simulink model "simscapeFuzzyComplete20Final"  (R2020b)
settings: Solver=FixedStepAuto  StartTime=0.0  StopTime=10  FixedStep=1e-5  RelTol=1e-1
InitFcn:
  | Param
values from neighbouring files (symbols this model uses):
  c = 3.5077E-3    (= 0.0035077)    [Param.m]
  g = 9.81    [Param.m]
  Jm = 3.2284E-3    (= 0.0032284)    [Param.m]
  K = 0.0274    [Param.m]
  L = 2.75E-3    (= 0.00275)    [Param.m]
  m = 0.051    [Param.m]
  R = 4    [Param.m]
undefined symbols (not defined in the file or in its folder): X, Y, Z
libraries: sm_lib x29, nesl_utility x10, fuzblock x2, simulink x2, pid_lib x2
(part 1 of 3)
settings Model: EnablePacing=on  Creator=HASSAN  LastModifiedBy=sara6
settings DebuggingCC: SFMachineParentedDataDiag=error
settings ExplorerConfigSet: InternalSimMechanicsExplorerSettings="<ExplorerConfiguration><canonicalview>default</canonicalview><AnimationSetting><BasePlaybackSpeed>1.0</BasePlaybackSpeed><PlaybackSpeedFactor>1.0</PlaybackSpeedFactor></AnimationSetting><TilePanel><TileInfo><Tiles Columns=\"1\" Count=\"1\" Rows=\"1\"><Column Weight=\"1\"/><Row Weight=\"1\"/><Tile Height=\"1\" Width=\"1\" X=\"0\" Y=\"0\"/></Tiles></TileInfo><SceneInfo><SceneViewer><BGColor><R>0.60000002384185791</R><G>0.60000002384185791</G><B>0.60000002384185791</B></BGColor><Camera><DoPerspective>off</DoPerspective><Position><X>0.124999998925166445</X><Y>0.0174999977718945862</Y><Z>1.04360001290421245</Z></Position><Center><X>0.124999998925166445</X><Y>0.0174999977718945862</Y><Z>0.0436000129042124485</Z></Center><Up><X>0</X><Y>1</Y><Z>-0</Z></Up><ViewLimDist>1</ViewLimDist><YLim>0.187288632229957203</YLim><XLim>0.154500006139278417</XLim></Camera></SceneViewer></SceneInfo></TilePanel><MechEditorPanel><Cameras/><GfxPanelCameraMap/><VideoCreator><PlaybackSpeedRatio>1.0</PlaybackSpeedRatio><FrameRate>30</FrameRate><VideoFormat>MPEG-4</VideoFormat><FrameSize>auto</FrameSize></VideoCreator></MechEditorPanel></ExplorerConfiguration>"

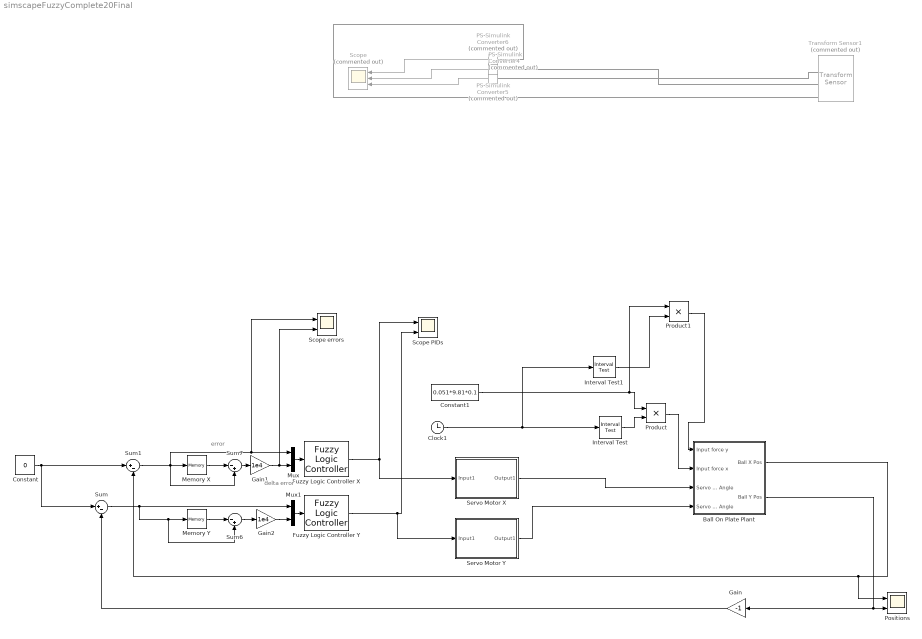
== system simscapeFuzzyComplete20Final ==
  note: delta error
  note: error
  Ball On Plate Plant : Subsystem
  Clock1 : Clock
  Constant : Constant  Value=0
  Constant1 : Constant  Value=0.051*9.81*0.1
  Fuzzy Logic Controller X : fuzblock/Fuzzy Logic  Controller  FIS='simpleFuzzy2.fis'  OutputSampleNumber=101  DataType=double  FuzzifiedInputs=off  RuleFiringStrengths=off  RuleOutputs=off  AggregatedOutputs=off  SimulateUsing=Code generation  OutOfRangeInputValueMessage=warning  NoRuleFiredMessage=warning  EmptyOutputFuzzySetMessage=warning
  Fuzzy Logic Controller Y : fuzblock/Fuzzy Logic  Controller  FIS='simpleFuzzy2.fis'  OutputSampleNumber=101  DataType=double  FuzzifiedInputs=off  RuleFiringStrengths=off  RuleOutputs=off  AggregatedOutputs=off  SimulateUsing=Code generation  OutOfRangeInputValueMessage=warning  NoRuleFiredMessage=warning  EmptyOutputFuzzySetMessage=warning
  Gain : Gain  Gain=-1
  Gain1 : Gain  Gain=1e4
  Gain2 : Gain  Gain=1e4
  Interval Test : simulink/Logic and Bit Operations/Interval Test  IntervalClosedRight=on  uplimit=0.2  IntervalClosedLeft=on  lowlimit=0.1  OutDataTypeStr=boolean
  Interval Test1 : simulink/Logic and Bit Operations/Interval Test  IntervalClosedRight=on  uplimit=0.2  IntervalClosedLeft=on  lowlimit=0.1  OutDataTypeStr=boolean
  Memory X : Memory
  Memory Y : Memory
  Mux : Mux  Inputs=2
  Mux1 : Mux  Inputs=2
  PS-Simulink Converter4 : nesl_utility/PS-Simulink Converter  Commented=on  PhysicalDomain=network_engine_domain  SubClassName=ps_output  LeftPortType=input  RightPortType=output  PseudoPeriodic=off  Frequencies=[]  Unit=inherit  AffineConversion=off
  PS-Simulink Converter5 : nesl_utility/PS-Simulink Converter  Commented=on  PhysicalDomain=network_engine_domain  SubClassName=ps_output  LeftPortType=input  RightPortType=output  PseudoPeriodic=off  Frequencies=[]  Unit=inherit  AffineConversion=off
  PS-Simulink Converter6 : nesl_utility/PS-Simulink Converter  Commented=on  PhysicalDomain=network_engine_domain  SubClassName=ps_output  LeftPortType=input  RightPortType=output  PseudoPeriodic=off  Frequencies=[]  Unit=inherit  AffineConversion=off
  Positions : Scope  NumInputPorts=2
  Product : Product
  Product1 : Product
  Scope : Scope  Commented=on  NumInputPorts=3
  Scope PIDs : Scope  NumInputPorts=2
  Scope errors : Scope  NumInputPorts=2
  Servo Motor X : Subsystem
  Servo Motor Y : Subsystem
  Sum : Sum  Inputs=|+-
  Sum1 : Sum  Inputs=|+-
  Sum6 : Sum  Inputs=|-+
  Sum7 : Sum  Inputs=|-+
  Transform Sensor1 : sm_lib/Frames and Transforms/Transform Sensor  Commented=on  MeasurementFrame=World  SenseAngle=off  SenseAxis=off  SenseAngle1=off  SenseAngle2=off  SenseAngle3=off  SenseQ=off  SenseR=off  SenseOmegaX=off  SenseOmegaY=off  SenseOmegaZ=off  SenseOmega1=off  SenseOmega2=off  SenseOmega3=off  SenseQDot=off  SenseRDot=off  SenseAlphaX=off  SenseAlphaY=off  SenseAlphaZ=off  SenseAlpha1=off  SenseAlpha2=off  SenseAlpha3=off  SenseQDDot=off  SenseRDDot=off  SenseX=on  SenseY=on  SenseZ=on  SenseRad=off  SenseAzim=off  SenseDist=off  SenseInc=off  SenseXDot=off  SenseYDot=off  SenseZDot=off  SenseRadDot=off  SenseAzimDot=off  SenseDistDot=off  SenseIncDot=off  SenseXDDot=off  SenseYDDot=off  SenseZDDot=off  SenseRadDDot=off  SenseAzimDDot=off  SenseDistDDot=off  SenseIncDDot=off
  wires:
  Constant/1 -> Sum1/1, Sum/1
  Sum1/1 -> Memory X/1, Scope errors/1, Mux/1, Sum7/2
  Ball On Plate Plant/1(Ball X Pos) -> Sum1/2, Positions/1
  Ball On Plate Plant/2(Ball Y Pos) -> Gain/1, Positions/2
  Clock1/1 -> Interval Test1/1, Interval Test/1
  PS-Simulink Converter4/1 -> Scope/3
  PS-Simulink Converter5/1 -> Scope/2
  PS-Simulink Converter6/1 -> Scope/1
  Sum/1 -> Mux1/1, Sum6/2, Memory Y/1
  Gain/1 -> Sum/2
  Product/1 -> Ball On Plate Plant/2(Input force x)
  Fuzzy Logic Controller X/1 -> Servo Motor X/1(Input1), Scope PIDs/1
  Fuzzy Logic Controller Y/1 -> Servo Motor Y/1(Input1), Scope PIDs/2
  Product1/1 -> Ball On Plate Plant/1(Input force y)
  Constant1/1 -> Product1/1, Product/1
  Interval Test1/1 -> Product1/2
  Interval Test/1 -> Product/2
  Memory Y/1 -> Sum6/1
  Memory X/1 -> Sum7/1
  Sum7/1 -> Gain1/1
  Gain1/1 -> Scope errors/2, Mux/2
  Gain2/1 -> Mux1/2
  Sum6/1 -> Gain2/1
  Mux/1 -> Fuzzy Logic Controller X/1
  Mux1/1 -> Fuzzy Logic Controller Y/1
  Servo Motor X/1(Output1) -> Ball On Plate Plant/3(Servo X Angle)
  Servo Motor Y/1(Output1) -> Ball On Plate Plant/4(Servo Y Angle)
  connections:
  Transform Sensor1/RConn2 -- PS-Simulink Converter4/LConn1
  Transform Sensor1/RConn3 -- PS-Simulink Converter5/LConn1
  Transform Sensor1/RConn4 -- PS-Simulink Converter6/LConn1
